simulink model "least_square"  (Simulink 10.3)
settings: Solver=ode45  StartTime=10  StopTime=20  RelTol=1e-3  AbsTol=1e-6
values from neighbouring files (symbols this model uses):
  As = 2    [sim_grad_norm.m]    (also in sim_grad_norm_2ordem.m = 0)
  DC = 1    [sim_grad_norm.m]    (also in sim_grad_norm_2ordem.m)
  kappa = 0    [sim_grad_norm.m]    (also in sim_grad_norm_2ordem.m = 1)
  lambda0 = 1    [sim_grad_norm.m]    (also in sim_grad_norm_2ordem.m)
  lambda1 = 2    [sim_grad_norm.m]    (also in sim_grad_norm_2ordem.m)
  P0 = 1*eye(4)    [sim_grad_norm.m]    (also in sim_grad_norm_2ordem.m)
  st = 0.01    [sim_grad_norm.m]    (also in sim_grad_norm_2ordem.m)
  theta0 = [0;0;0;0]    [sim_grad_norm.m]    (also in sim_grad_norm_2ordem.m)
  theta_star = theta_star3    [sim_grad_norm.m]    (also in sim_grad_norm_2ordem.m = theta_star1)
  ws = 0.1*pi    (= 0.314159265359)    [sim_grad_norm.m]    (also in sim_grad_norm_2ordem.m = 3.14159265359)
libraries: cstblocks x1
settings Model: LogicAnalyzerSignalOrdering=a3ae0bb2-648e-49cc-b532-501527ad276f,919e012d-1cd0-4a05-ae56-aa165e610728,b400014a-40bf-49f6-9e38-b7c144e10992,70793da9-eb15-4f57-99ee-5707dcc79d9b,2ef5c575-fcfa-49cc-b545-e8a8b41c0ea7,fea41da3-d57e-44aa-96d4-4ceda414349f,8f7b36af-7405-431b-9f2e-81f8b2f0f1ee  Creator=Ramon  LastModifiedBy=linco  MultithreadedSim=on
settings SolverCC: AutoScaleAbsTol=off
settings DataIOCC: SaveOutput=off  SaveTime=off
settings OptimizationCC: BlockReduction=off  BooleanDataType=off  InitFltsAndDblsToZero=on
settings DebuggingCC: SaveWithParameterizedLinksMsg=none  SignalResolutionControl=TryResolveAllWithWarning  MultiTaskDSMMsg=warning  MultiTaskCondExecSysMsg=none
settings HardwareCC: TargetUnknown=on
settings RTWCC: TemplateMakefile=grt_vc.tmf

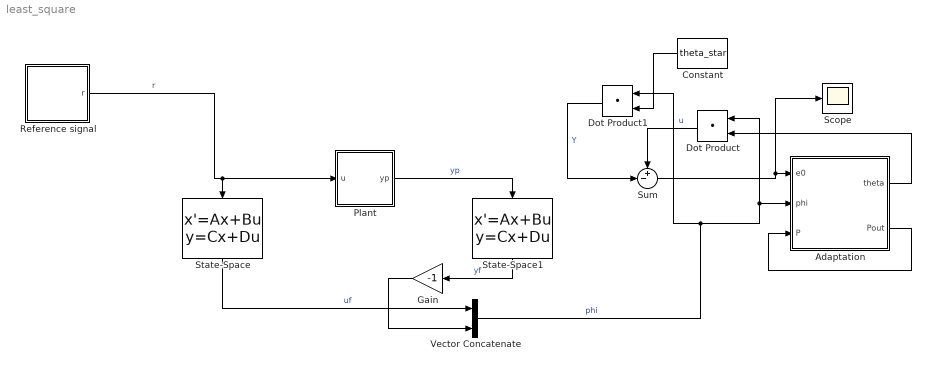
== system least_square ==
  Adaptation : Subsystem
  Constant : Constant  Value=theta_star
  Dot Product : DotProduct  InputSameDT=on  OutDataTypeStr=Inherit: Inherit via internal rule
  Dot Product1 : DotProduct  InputSameDT=on  OutDataTypeStr=Inherit: Inherit via internal rule
  Gain : Gain  Gain=-1
  Plant : Subsystem
  Reference signal : Subsystem
  Scope : Scope
  State-Space : StateSpace  A=[0 1; -lambda0 -lambda1]  B=[0; 1]  C=[1 0;0 1]  D=[0; 0]  InitialCondition=0
  State-Space1 : StateSpace  A=[0 1; -lambda0 -lambda1]  B=[0; 1]  C=[1 0;0 1]  D=[0; 0]  InitialCondition=0
  Sum : Sum  Inputs=+-|
  Vector Concatenate : Concatenate
  wires:
  Adaptation/1(theta) -> Dot Product/2
  Vector Concatenate/1 -> Adaptation/2(phi), Dot Product/1, Dot Product1/1  "phi"
  Reference signal/1(r) -> State-Space/1, Plant/1(u)  "r"
  Plant/1(yp) -> State-Space1/1  "yp"
  State-Space1/1 -> Gain/1  "yf"
  State-Space/1 -> Vector Concatenate/1  "uf"
  Gain/1 -> Vector Concatenate/2
  Sum/1 -> Scope/1, Adaptation/1(e0)
  Dot Product/1 -> Sum/1  "u"
  Constant/1 -> Dot Product1/2
  Dot Product1/1 -> Sum/2  "Y"
  Adaptation/2(Pout) -> Adaptation/3(P)

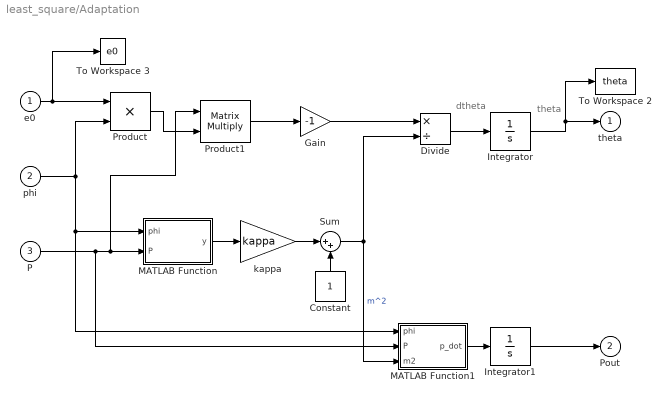
== system least_square/Adaptation ==
  note: theta
  note: dtheta
  e0 : Inport  PortDimensions=1
  phi : Inport  Port=2
  P : Inport  Port=3
  Constant : Constant
  Divide : Product  Inputs=*/
  Gain : Gain  Gain=-1
  Integrator : Integrator  InitialCondition=theta0
  Integrator1 : Integrator  InitialCondition=P0
  MATLAB Function : MATLAB Function  TreatAsAtomicUnit=on
  MATLAB Function1 : MATLAB Function  TreatAsAtomicUnit=on
  Product : Product  InputSameDT=on  RndMeth=Zero  SaturateOnIntegerOverflow=on  OutDataTypeStr=Inherit: Same as first input
  Product1 : Product  Multiplication=Matrix(*)
  Sum : Sum  Inputs=|++
  To Workspace 2 : ToWorkspace  VariableName=theta  SampleTime=st
  To Workspace 3 : ToWorkspace  VariableName=e0  SampleTime=st
  kappa : Gain  Gain=kappa  SaturateOnIntegerOverflow=on  OutDataTypeStr=Inherit: Same as input  ParamDataTypeStr=Inherit: Same as input
  theta : Outport  InitialOutput=0  VectorParamsAs1DForOutWhenUnconnected=off
  Pout : Outport  Port=2  InitialOutput=0  VectorParamsAs1DForOutWhenUnconnected=off
  wires:
  Integrator/1 -> To Workspace 2/1, theta/1
  Divide/1 -> Integrator/1
  phi/1 -> MATLAB Function1/1(phi), MATLAB Function/1(phi), Product/2
  e0/1 -> Product/1, To Workspace 3/1
  Product1/1 -> Gain/1
  Product/1 -> Product1/2
  MATLAB Function/1(y) -> kappa/1
  Constant/1 -> Sum/2
  kappa/1 -> Sum/1
  Sum/1 -> MATLAB Function1/3(m2), Divide/2  "m^2"
  Integrator1/1 -> Pout/1
  P/1 -> MATLAB Function1/2(P), Product1/1, MATLAB Function/2(P)
  Gain/1 -> Divide/1
  MATLAB Function1/1(p_dot) -> Integrator1/1

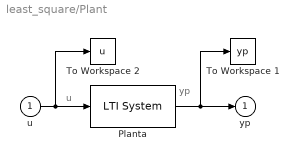
== system least_square/Plant ==
  note: yp
  note: u
  u : Inport
  Planta : cstblocks/LTI System  sys=P  IC=x0
  To Workspace 1 : ToWorkspace  VariableName=yp  SampleTime=st
  To Workspace 2 : ToWorkspace  VariableName=u  SampleTime=st
  yp : Outport  InitialOutput=0  VectorParamsAs1DForOutWhenUnconnected=off
  wires:
  u/1 -> To Workspace 2/1, Planta/1
  Planta/1 -> yp/1, To Workspace 1/1

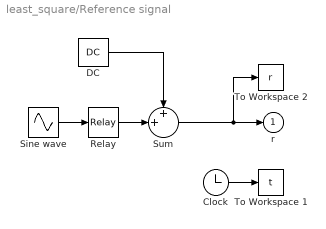
== system least_square/Reference signal ==
  Clock : Clock
  DC : Constant  Value=DC
  Relay : Relay  OnOutputValue=As  OffOutputValue=-As
  Sine wave : Sin  Frequency=ws  SampleTime=0
  Sum : Sum  Inputs=++|  InputSameDT=on  SaturateOnIntegerOverflow=on  OutDataTypeStr=Inherit: Same as first input
  To Workspace 1 : ToWorkspace  VariableName=t  SampleTime=st
  To Workspace 2 : ToWorkspace  VariableName=r  SampleTime=st
  r : Outport  InitialOutput=0  VectorParamsAs1DForOutWhenUnconnected=off
  wires:
  DC/1 -> Sum/1
  Sum/1 -> r/1, To Workspace 2/1
  Clock/1 -> To Workspace 1/1
  Sine wave/1 -> Relay/1
  Relay/1 -> Sum/2

== matlab function Adaptation/MATLAB Function1 ==
  data: phi input double; p_dot output double; P input double; m2 input double
function p_dot = fcn(phi,P,m2)

p_dot = -(P*phi*phi'*P)/m2;

== matlab function Adaptation/MATLAB Function ==
  data: phi input double; y output double; P input double
function y = fcn(phi,P)

y = phi'*P*phi;
